simulink model "torque_pi_controller_discrete"  (R2023b)
settings: Solver=VariableStepAuto  StartTime=0.0  StopTime=3.5  FixedStep=0.001  RelTol=1e-10
values from neighbouring files (symbols this model uses):
  K = 1.339    [torque_PI_integral_algorithm.m]    (also in torque_PI_tuning.m; torque_model.m = 1.32)
  Kp = pid.Kp    [torque_PI_integral_algorithm.m]
  Ti = pid.Ti    [torque_PI_integral_algorithm.m]
settings Model: Creator=paoli  LastModifiedBy=kiraa

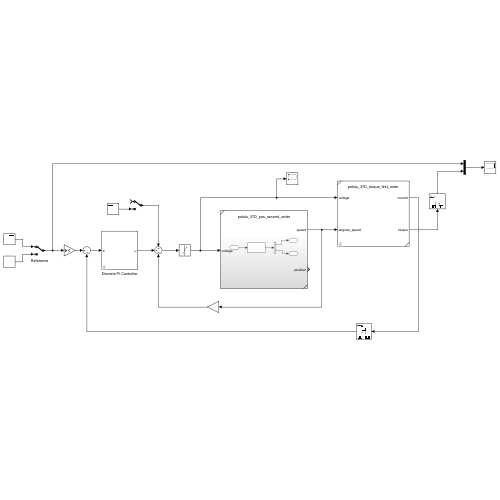
[thumbnail: Simulink's stored preview of the top-level diagram]
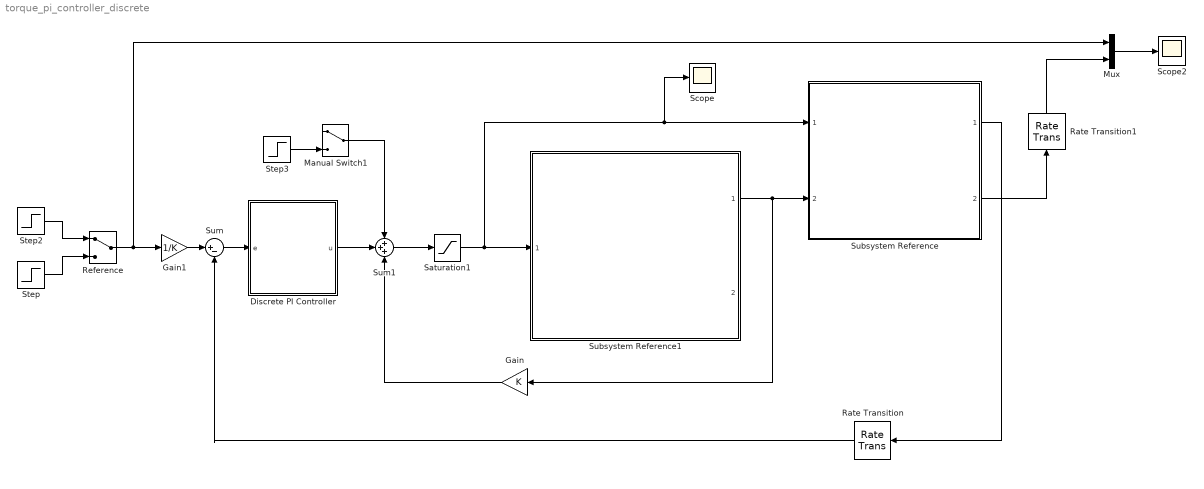
== system torque_pi_controller_discrete ==
  Discrete PI Controller : Subsystem  mask{Ts=0.005}
  Gain : Gain  Gain=K
  Gain1 : Gain  Gain=1/K
  Manual Switch1 : ManualSwitch
  Mux : Mux  Inputs=2
  Rate Transition : RateTransition  OutPortSampleTime=Ts
  Rate Transition1 : RateTransition  OutPortSampleTime=Ts
  Reference : ManualSwitch
  Saturation1 : Saturate  UpperLimit=12  LowerLimit=-12
  Scope : Scope
  Scope2 : Scope
  Step : Step  Time=2  Before=1  After=0  SampleTime=0
  Step2 : Step  Time=0  After=0.15  SampleTime=0
  Step3 : Step  Time=2  After=-0.1  SampleTime=0
  Subsystem Reference : Subsystem  ReferencedSubsystem=pololu_37D_torque_first_order  L=2.3e-3  R=1.7  K=1.339
  Subsystem Reference1 : Subsystem  ReferencedSubsystem=pololu_37D_pos_second_order
  Sum : Sum  Inputs=|+-
  Sum1 : Sum  Inputs=+++
  wires:
  Subsystem Reference/2 -> Rate Transition1/1
  Gain1/1 -> Sum/1
  Subsystem Reference1/1 -> Subsystem Reference/2, Gain/1
  Sum1/1 -> Saturation1/1
  Discrete PI Controller/1(u) -> Sum1/2
  Saturation1/1 -> Scope/1, Subsystem Reference/1, Subsystem Reference1/1
  Sum/1 -> Discrete PI Controller/1(e)
  Step/1 -> Reference/2
  Step2/1 -> Reference/1
  Reference/1 -> Mux/1, Gain1/1
  Mux/1 -> Scope2/1
  Subsystem Reference/1 -> Rate Transition/1
  Step3/1 -> Manual Switch1/2
  Manual Switch1/1 -> Sum1/1
  Rate Transition/1 -> Sum/2
  Rate Transition1/1 -> Mux/2
  Gain/1 -> Sum1/3

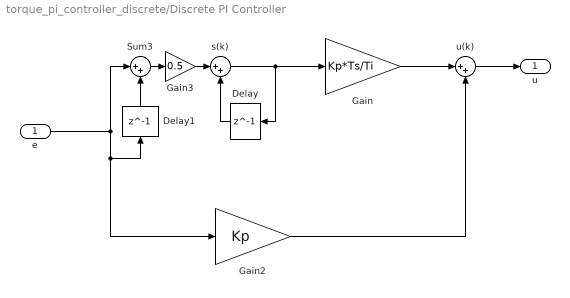
== system torque_pi_controller_discrete/Discrete PI Controller ==
  e : Inport  SampleTime=Ts
  Delay : Delay  DelayLength=1  InitialCondition=0  UseCircularBuffer=on
  Delay1 : Delay  DelayLength=1  InitialCondition=0  UseCircularBuffer=on
  Gain : Gain  Gain=Kp*Ts/Ti
  Gain2 : Gain  Gain=Kp
  Gain3 : Gain  Gain=0.5
  Sum3 : Sum  Inputs=|++
  s(k) : Sum  Inputs=|++
  u(k) : Sum  Inputs=|++
  u : Outport  SampleTime=Ts
  wires:
  e/1 -> Gain2/1, Delay1/1, Sum3/1
  Gain/1 -> u(k)/1
  Gain2/1 -> u(k)/2
  Delay/1 -> s(k)/2
  s(k)/1 -> Gain/1, Delay/1
  Delay1/1 -> Sum3/2
  Sum3/1 -> Gain3/1
  Gain3/1 -> s(k)/1
  u(k)/1 -> u/1
